simulink model "pixhawkController"  (R2016b)
settings: Solver=FixedStepDiscrete  StartTime=0.0  StopTime=inf  FixedStep=0.01  RelTol=1e-3  EnableMultiTasking=on
undefined symbols (not defined in the file): dt_pixhawk, KiPitchAttitude, KiPitchRate, KiRollAttitude, KiRollRate, KiYawRate, KpPitchAttitude, KpPitchRate, KpRollAttitude, KpRollRate, KpYawRate, PX4_TUNE_ENUM, RGBLED_COLOR_ENUM, RGBLED_MODE_ENUM
libraries: xpcutilitieslib x32, simulink x11, pixhawk_slib_sensors_actuators x8, pixhawk_slib_ADC_serial x2
settings Model: Creator=darenlee  LastModifiedBy=ers
settings DataIOCC: LimitDataPoints=on  SaveFormat=StructureWithTime
settings OptimizationCC: DefaultParameterBehavior=Inlined  LifeSpan=1  MaxStackSize=64
settings DebuggingCC: AllowSymbolicDim=off  SFUnexpectedBacktrackingDiag=warning  SFNoUnconditionalDefaultTransitionDiag=warning  SFExecutionAtInitializationDiag=none
settings HardwareCC: ProdBitPerPointer=32  ProdBitPerSizeT=32  ProdBitPerPtrDiffT=32  ProdLargestAtomicInteger=Long  ProdLargestAtomicFloat=Double  ProdIntDivRoundTo=Undefined  ProdWordSize=32  ProdHWDeviceType=ARM Compatible->ARM Cortex
settings ModelReferenceCC: PropagateSignalLabelsOutOfModel=off
settings RTWCC: SystemTargetFile=ert.tlc  HardwareBoard=Pixhawk PX4  TLCOptions=-aInlineSetEventsForThisBaseRateFcn=TLC_FALSE -aSuppressMultiTaskScheduler=TLC_FALSE -aRateBasedStepFcn=0  TemplateMakefile=ert_default_tmf  Description=Embedded Coder  GenerateReport=on  Toolchain=Pixhawk Toolchain  IncludeHyperlinkInReport=on  LaunchReport=on  GenerateTraceInfo=on  GenerateTraceReport=on  GenerateTraceReportSl=on  GenerateTraceReportSf=on  GenerateTraceReportEml=on
settings CodeAppCC: IgnoreCustomStorageClasses=off
settings ERTTargetCC: ExtModeTransport=1  ExtModeMexFile=ext_serial_win32_comm  ExtModeMexArgs=1 11 115200 5  ERTCustomFileTemplate=PX4_codertarget_file_process.tlc  ConvertIfToSwitch=off  SuppressUnreachableDefaultCases=off
settings ConfigComp: CovMetricSettings=dw  CovHtmlReporting=on  CovSaveCumulativeToWorkspaceVar=on  CovSaveSingleToWorkspaceVar=on  CovExternalEMLEnable=off

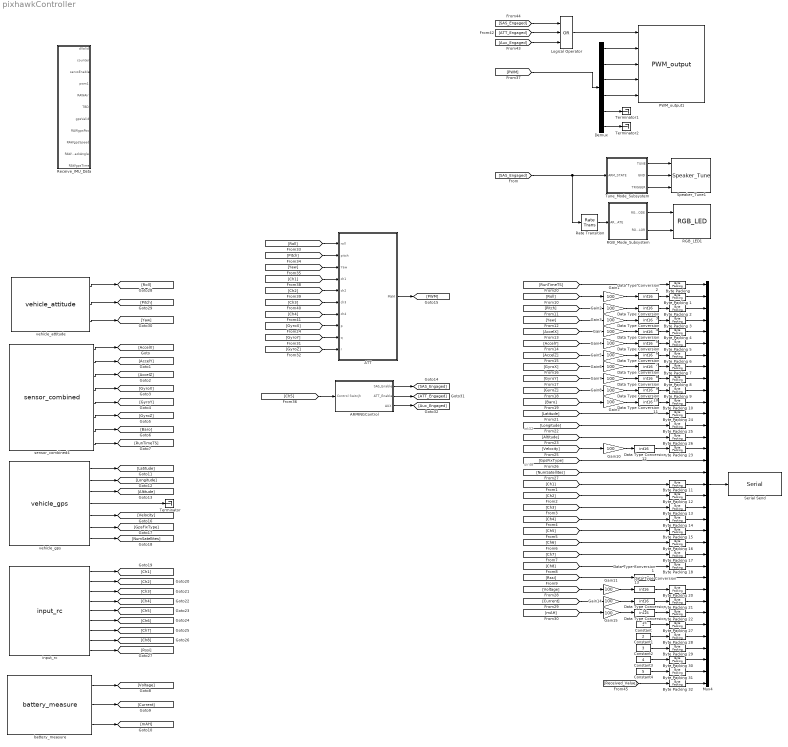
== system pixhawkController ==
  note: uint8
  note: int32
  ARMINGControl : Subsystem
  ATT : Subsystem
  Byte Packing {,1..18,20..32} (32 alike) : xpcutilitieslib/Byte Packing 
  Constant : Constant  OutDataTypeStr=int16
  Constant1 : Constant  Value=2  OutDataTypeStr=int16
  Constant2 : Constant  Value=3  OutDataTypeStr=int16
  Constant3 : Constant  Value=4  OutDataTypeStr=int16
  Constant4 : Constant  Value=5  OutDataTypeStr=int16
  Data Type Conversion1 : DataTypeConversion  OutDataTypeStr=uint8
  Data Type Conversion{2..15} (14 alike) : DataTypeConversion  OutDataTypeStr=int16
  Demux : Demux  Outputs=6
  Gain{,1..11,14..15} (14 alike) : Gain  Gain=100
  Logical Operator : Logic  Operator=OR  Inputs=3  AllPortsSameDT=off  OutDataTypeStr=boolean
  Mux4 : Mux  Inputs=35
  PWM_output1 : pixhawk_slib_sensors_actuators/PWM_output  pwm_rate=50Hz  show_pwm1=on  show_pwm2=on  show_pwm3=on  show_pwm4=on  show_pwm5=off  show_pwm6=off  show_pwm7=off  show_pwm8=off
  RGB_LED1 : pixhawk_slib_sensors_actuators/RGB_LED
  RGB_Mode_Subsystem : Subsystem
  Rate Transition : RateTransition  OutPortSampleTime=1/2
  Receive_IMU_Data : Subsystem
  Serial Send : pixhawk_slib_ADC_serial/Serial  DeviceName=/dev/ttyS5  ReadOrWrite=Writing  BaudRateStr=115200  block=off  WriteStatus=on  Terminator=off  Header=on  NumBytesRead=4  TerminatorChar=\n  HeaderData=[ uint8( hex2dec( '41' ) ), uint8( hex2dec( '42' ) ), uint8( hex2dec( '43' ) ), uint8( hex2dec( '41' ) ) ]  SimulateUsing=Code generation
  Speaker_Tune1 : pixhawk_slib_sensors_actuators/Speaker_Tune
  Terminator : Terminator
  Terminator1 : Terminator
  Terminator2 : Terminator
  Tune_Mode_Subsystem : Subsystem
  battery_measure : pixhawk_slib_sensors_actuators/battery_measure  SampleTime=dt_pixhawk  VoltageOut=on  VoltageFilteredOut=off  CurrentOut=on  mAH_Out=on  TimeStamp=off
  input_rc : pixhawk_slib_sensors_actuators/input_rc  sampletime=dt_pixhawk  channel1=on  channel2=on  channel3=on  channel4=on  channel5=on  channel6=on  channel7=on  channel8=on  ch_count=off  rssi=on  rc_failsafe=off  rc_lost=off  rc_inputsource=off
  sensor_combined4 : pixhawk_slib_sensors_actuators/sensor_combined  sampletime=dt_pixhawk  show_mag=off  show_acc=on  show_gyro=on  show_baro=on  show_ts=on
  vehicle_attitude : pixhawk_slib_sensors_actuators/vehicle_attitude  sampletime=dt_pixhawk  show_r=on  show_p=on  show_y=on  show_q=off
  vehicle_gps : pixhawk_slib_sensors_actuators/vehicle_gps  sampletime=1/100  show_ts_pos=off  show_alt=on  show_ts_gps=off  show_vel=on  show_fixtype=on  show_numsat=on
  wires:
  sensor_combined4/8 -> [RunTimeTS]
  battery_measure/1 -> [Voltage]
  battery_measure/3 -> [mAH]
  battery_measure/2 -> [Current]
  vehicle_gps/2 -> [Longitude]
  vehicle_gps/1 -> [Latitude]
  vehicle_gps/3 -> [Altitude]
  input_rc/2 -> [Ch2]
  input_rc/3 -> [Ch3]
  input_rc/6 -> [Ch6]
  input_rc/8 -> [Ch8]
  input_rc/7 -> [Ch7]
  input_rc/5 -> [Ch5]
  input_rc/4 -> [Ch4]
  input_rc/1 -> [Ch1]
  input_rc/9 -> [Rssi]
  vehicle_attitude/1 -> [Roll]
  vehicle_attitude/2 -> [Pitch]
  vehicle_attitude/3 -> [Yaw]
  vehicle_gps/6 -> [GpsFixType]
  vehicle_gps/5 -> [Velocity]
  vehicle_gps/7 -> [NumSatellites]
  vehicle_gps/4 -> Terminator/1
  "Byte Packing "/1 -> Mux4/1
  [Pitch] -> Gain2/1
  Mux4/1 -> Serial Send/1
  Byte Packing 1/1 -> Mux4/2
  Byte Packing 2/1 -> Mux4/3
  Byte Packing 3/1 -> Mux4/4
  sensor_combined4/4 -> [GyroX]
  sensor_combined4/3 -> [AccelZ]
  sensor_combined4/5 -> [GyroY]
  sensor_combined4/2 -> [AccelY]
  sensor_combined4/6 -> [GyroZ]
  sensor_combined4/7 -> [Baro]
  sensor_combined4/1 -> [AccelX]
  [AccelX] -> Gain/1
  [AccelY] -> Gain4/1
  [AccelZ] -> Gain5/1
  [GyroX] -> Gain6/1
  [GyroY] -> Gain7/1
  [GyroZ] -> Gain8/1
  [Baro] -> Gain9/1
  [Ch1] -> Byte Packing 11/1
  [Ch2] -> Byte Packing 12/1
  [Ch3] -> Byte Packing 13/1
  [Ch4] -> Byte Packing 14/1
  [Ch5] -> Byte Packing 15/1
  [Ch6] -> Byte Packing 16/1
  [Ch7] -> Byte Packing 17/1
  [Ch8] -> Byte Packing 18/1
  [Rssi] -> Data Type Conversion1/1
  [mAH] -> Gain15/1
  [Current] -> Gain14/1
  [Voltage] -> Gain11/1
  [RunTimeTS] -> "Byte Packing "/1
  [Roll] -> Gain1/1
  Data Type Conversion3/1 -> Byte Packing 2/1
  [Yaw] -> Gain3/1
  Data Type Conversion4/1 -> Byte Packing 3/1
  Data Type Conversion2/1 -> Byte Packing 1/1
  Gain1/1 -> Data Type Conversion2/1
  Gain2/1 -> Data Type Conversion3/1
  Gain3/1 -> Data Type Conversion4/1
  Gain/1 -> Data Type Conversion5/1
  Gain4/1 -> Data Type Conversion6/1
  Gain5/1 -> Data Type Conversion7/1
  Gain6/1 -> Data Type Conversion8/1
  Gain7/1 -> Data Type Conversion9/1
  Gain8/1 -> Data Type Conversion10/1
  Gain9/1 -> Data Type Conversion11/1
  Data Type Conversion5/1 -> Byte Packing 4/1
  Data Type Conversion6/1 -> Byte Packing 5/1
  Data Type Conversion7/1 -> Byte Packing 6/1
  Data Type Conversion8/1 -> Byte Packing 7/1
  Data Type Conversion9/1 -> Byte Packing 8/1
  Data Type Conversion10/1 -> Byte Packing 9/1
  Data Type Conversion11/1 -> Byte Packing 10/1
  [Velocity] -> Gain10/1
  Gain10/1 -> Data Type Conversion12/1
  Data Type Conversion12/1 -> Byte Packing 23/1
  [Latitude] -> Byte Packing 24/1
  [Longitude] -> Byte Packing 25/1
  [Altitude] -> Byte Packing 26/1
  [GpsFixType] -> Mux4/16
  [NumSatellites] -> Mux4/17
  Gain11/1 -> Data Type Conversion13/1
  Gain14/1 -> Data Type Conversion14/1
  Gain15/1 -> Data Type Conversion15/1
  Data Type Conversion13/1 -> Byte Packing 20/1
  Data Type Conversion14/1 -> Byte Packing 21/1
  Data Type Conversion15/1 -> Byte Packing 22/1
  Byte Packing 4/1 -> Mux4/5
  Byte Packing 5/1 -> Mux4/6
  Byte Packing 6/1 -> Mux4/7
  Byte Packing 7/1 -> Mux4/8
  Byte Packing 8/1 -> Mux4/9
  Byte Packing 9/1 -> Mux4/10
  Byte Packing 10/1 -> Mux4/11
  Byte Packing 25/1 -> Mux4/13
  Byte Packing 26/1 -> Mux4/14
  Byte Packing 24/1 -> Mux4/12
  Byte Packing 23/1 -> Mux4/15
  Byte Packing 11/1 -> Mux4/18
  Byte Packing 12/1 -> Mux4/19
  Byte Packing 13/1 -> Mux4/20
  Byte Packing 14/1 -> Mux4/21
  Byte Packing 15/1 -> Mux4/22
  Byte Packing 16/1 -> Mux4/23
  Byte Packing 17/1 -> Mux4/24
  Byte Packing 18/1 -> Mux4/25
  Data Type Conversion1/1 -> Mux4/26
  Byte Packing 20/1 -> Mux4/27
  Byte Packing 21/1 -> Mux4/28
  Byte Packing 22/1 -> Mux4/29
  Constant/1 -> Byte Packing 27/1
  Byte Packing 32/1 -> Mux4/35
  Byte Packing 27/1 -> Mux4/30
  Byte Packing 30/1 -> Mux4/33
  Byte Packing 28/1 -> Mux4/31
  Byte Packing 31/1 -> Mux4/34
  Byte Packing 29/1 -> Mux4/32
  Constant1/1 -> Byte Packing 28/1
  Constant2/1 -> Byte Packing 29/1
  Constant3/1 -> Byte Packing 30/1
  Constant4/1 -> Byte Packing 31/1
  RGB_Mode_Subsystem/1(RGB_MODE) -> RGB_LED1/1
  RGB_Mode_Subsystem/2(RGB_COLOR) -> RGB_LED1/2
  Tune_Mode_Subsystem/1(TUNE) -> Speaker_Tune1/1
  Tune_Mode_Subsystem/2(GND) -> Speaker_Tune1/2
  Tune_Mode_Subsystem/3(TRIGGER) -> Speaker_Tune1/3
  [SAS_Engaged] -> Tune_Mode_Subsystem/1(ARM_STATE), Rate Transition/1
  ATT/1(PWM) -> [PWM]
  [Roll] -> ATT/1(roll)
  [Pitch] -> ATT/2(pitch)
  [Yaw] -> ATT/3(Yaw)
  [Ch4] -> ATT/7(ch4)
  [Ch3] -> ATT/6(ch3)
  [Ch2] -> ATT/5(ch2)
  [Ch1] -> ATT/4(ch1)
  [GyroX] -> ATT/8(p)
  [GyroY] -> ATT/9(q)
  [GyroZ] -> ATT/10(r)
  Demux/3 -> PWM_output1/4
  Demux/4 -> PWM_output1/5
  Demux/2 -> PWM_output1/3
  Demux/1 -> PWM_output1/2
  [Ch5] -> ARMINGControl/1(Control Switcjh)
  ARMINGControl/1(SAS_Enable) -> [SAS_Engaged]
  ARMINGControl/2(ATT_Enable) -> [ATT_Engaged]
  ARMINGControl/3(AUX) -> [Aux_Engaged]
  [SAS_Engaged] -> Logical Operator/1
  [ATT_Engaged] -> Logical Operator/2
  [Aux_Engaged] -> Logical Operator/3
  Logical Operator/1 -> PWM_output1/1
  [Received_Value] -> Byte Packing 32/1
  [PWM] -> Demux/1
  Demux/5 -> Terminator1/1
  Demux/6 -> Terminator2/1
  Rate Transition/1 -> RGB_Mode_Subsystem/1(ARM_STATE)

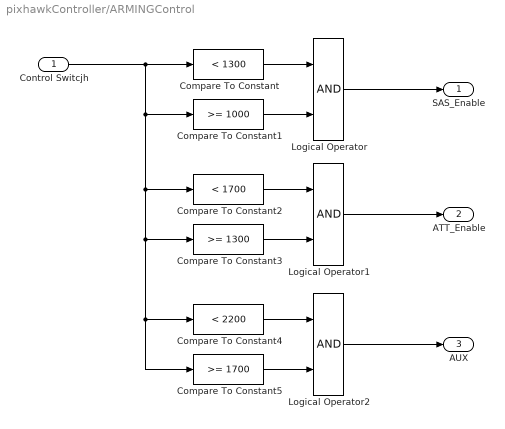
== system pixhawkController/ARMINGControl ==
  Control Switcjh : Inport
  Compare To Constant : simulink/Logic and Bit Operations/Compare To Constant  relop=<  const=1300  OutDataTypeStr=boolean
  Compare To Constant1 : simulink/Logic and Bit Operations/Compare To Constant  relop=>=  const=1000  OutDataTypeStr=boolean
  Compare To Constant2 : simulink/Logic and Bit Operations/Compare To Constant  relop=<  const=1700  OutDataTypeStr=boolean
  Compare To Constant3 : simulink/Logic and Bit Operations/Compare To Constant  relop=>=  const=1300  OutDataTypeStr=boolean
  Compare To Constant4 : simulink/Logic and Bit Operations/Compare To Constant  relop=<  const=2200  OutDataTypeStr=boolean
  Compare To Constant5 : simulink/Logic and Bit Operations/Compare To Constant  relop=>=  const=1700  OutDataTypeStr=boolean
  Logical Operator : Logic  AllPortsSameDT=off  OutDataTypeStr=boolean
  Logical Operator1 : Logic  AllPortsSameDT=off  OutDataTypeStr=boolean
  Logical Operator2 : Logic  AllPortsSameDT=off  OutDataTypeStr=boolean
  SAS_Enable : Outport
  ATT_Enable : Outport  Port=2
  AUX : Outport  Port=3
  wires:
  Control Switcjh/1 -> Compare To Constant5/1, Compare To Constant4/1, Compare To Constant3/1, Compare To Constant2/1, Compare To Constant1/1, Compare To Constant/1
  Compare To Constant/1 -> Logical Operator/1
  Compare To Constant1/1 -> Logical Operator/2
  Logical Operator/1 -> SAS_Enable/1
  Compare To Constant2/1 -> Logical Operator1/1
  Compare To Constant3/1 -> Logical Operator1/2
  Logical Operator1/1 -> ATT_Enable/1
  Compare To Constant4/1 -> Logical Operator2/1
  Compare To Constant5/1 -> Logical Operator2/2
  Logical Operator2/1 -> AUX/1

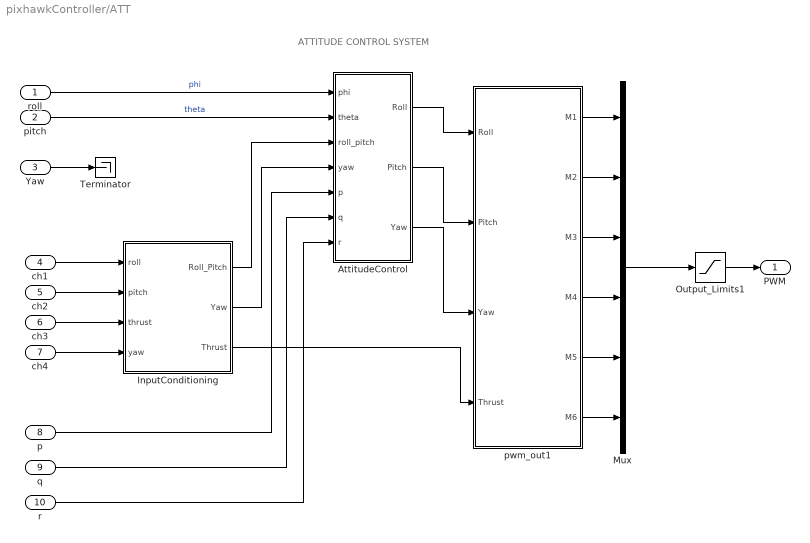
== system pixhawkController/ATT ==
  note: ATTITUDE CONTROL SYSTEM
  roll : Inport  OutDataTypeStr=single  PortDimensions=1
  pitch : Inport  Port=2  PortDimensions=1
  Yaw : Inport  Port=3  PortDimensions=1
  ch1 : Inport  Port=4  OutDataTypeStr=uint16  PortDimensions=1
  ch2 : Inport  Port=5  OutDataTypeStr=uint16  PortDimensions=1
  ch3 : Inport  Port=6  OutDataTypeStr=uint16  PortDimensions=1
  ch4 : Inport  Port=7  OutDataTypeStr=uint16  PortDimensions=1
  p : Inport  Port=8  PortDimensions=1
  q : Inport  Port=9  PortDimensions=1
  r : Inport  Port=10  PortDimensions=1
  AttitudeControl : Subsystem
  InputConditioning : Subsystem
  Mux : Mux  Inputs=6
  Output_Limits1 : Saturate  UpperLimit=2000  LowerLimit=1000
  Terminator : Terminator
  pwm_out1 : MATLAB Function  TreatAsAtomicUnit=on  SystemSampleTime=dt_pixhawk
  PWM : Outport  PortDimensions=6
  wires:
  Mux/1 -> Output_Limits1/1
  Output_Limits1/1 -> PWM/1
  InputConditioning/3(Thrust) -> pwm_out1/4(Thrust)
  roll/1 -> AttitudeControl/1(phi)  "phi"
  pitch/1 -> AttitudeControl/2(theta)  "theta"
  InputConditioning/1(Roll_Pitch) -> AttitudeControl/3(roll_pitch)
  InputConditioning/2(Yaw) -> AttitudeControl/4(yaw)
  p/1 -> AttitudeControl/5(p)
  q/1 -> AttitudeControl/6(q)
  r/1 -> AttitudeControl/7(r)
  AttitudeControl/1(Roll) -> pwm_out1/1(Roll)
  AttitudeControl/2(Pitch) -> pwm_out1/2(Pitch)
  AttitudeControl/3(Yaw) -> pwm_out1/3(Yaw)
  ch1/1 -> InputConditioning/1(roll)
  ch2/1 -> InputConditioning/2(pitch)
  ch4/1 -> InputConditioning/4(yaw)
  ch3/1 -> InputConditioning/3(thrust)
  Yaw/1 -> Terminator/1
  pwm_out1/4(M4) -> Mux/4
  pwm_out1/3(M3) -> Mux/3
  pwm_out1/2(M2) -> Mux/2
  pwm_out1/1(M1) -> Mux/1
  pwm_out1/5(M5) -> Mux/5
  pwm_out1/6(M6) -> Mux/6

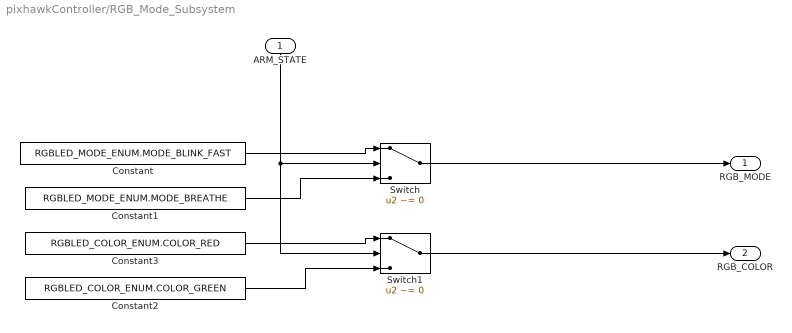
== system pixhawkController/RGB_Mode_Subsystem ==
  ARM_STATE : Inport
  Constant : Constant  Value=RGBLED_MODE_ENUM.MODE_BLINK_FAST  OutDataTypeStr=Enum: RGBLED_MODE_ENUM
  Constant1 : Constant  Value=RGBLED_MODE_ENUM.MODE_BREATHE  OutDataTypeStr=Enum: RGBLED_MODE_ENUM
  Constant2 : Constant  Value=RGBLED_COLOR_ENUM.COLOR_GREEN  OutDataTypeStr=Enum: RGBLED_COLOR_ENUM
  Constant3 : Constant  Value=RGBLED_COLOR_ENUM.COLOR_RED  OutDataTypeStr=Enum: RGBLED_COLOR_ENUM
  Switch : Switch  Criteria=u2 ~= 0  Threshold=1500  SampleTime=1/2
  Switch1 : Switch  Criteria=u2 ~= 0  Threshold=1500  SampleTime=1/2
  RGB_MODE : Outport
  RGB_COLOR : Outport  Port=2
  wires:
  ARM_STATE/1 -> Switch1/2, Switch/2
  Constant/1 -> Switch/1
  Constant1/1 -> Switch/3
  Switch/1 -> RGB_MODE/1
  Constant3/1 -> Switch1/1
  Constant2/1 -> Switch1/3
  Switch1/1 -> RGB_COLOR/1

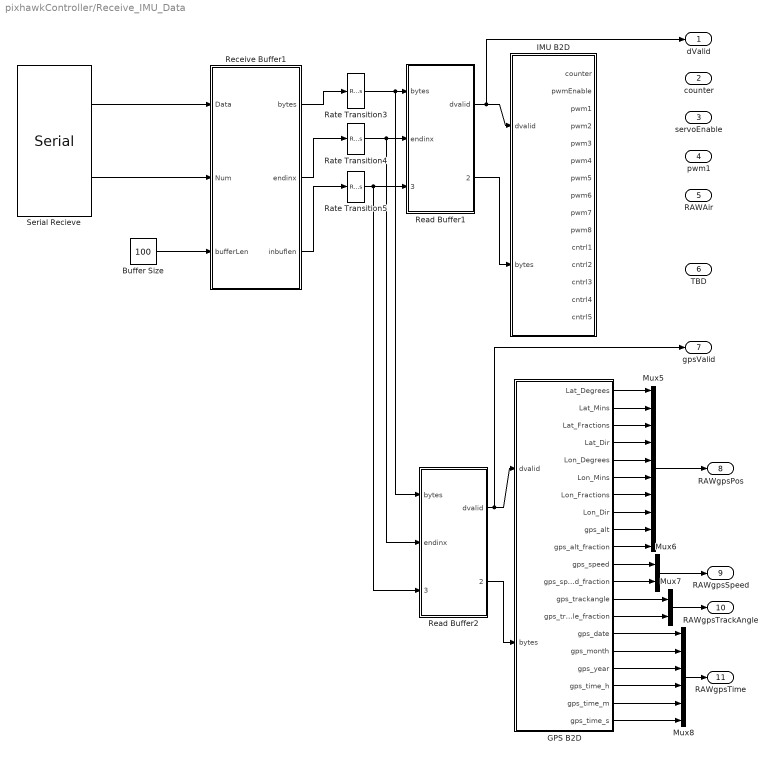
== system pixhawkController/Receive_IMU_Data ==
  Buffer Size : Constant  Value=100
  GPS B2D : MATLAB Function  TreatAsAtomicUnit=on
  IMU B2D : MATLAB Function  TreatAsAtomicUnit=on
  Mux5 : Mux  Inputs=10
  Mux6 : Mux  Inputs=2
  Mux7 : Mux  Inputs=2
  Mux8 : Mux  Inputs=6
  Rate Transition3 : RateTransition  OutPortSampleTime=dt
  Rate Transition4 : RateTransition  OutPortSampleTime=dt
  Rate Transition5 : RateTransition  OutPortSampleTime=dt
  Read Buffer1 : MATLAB Function  TreatAsAtomicUnit=on
  Read Buffer2 : MATLAB Function  TreatAsAtomicUnit=on
  Receive Buffer1 : MATLAB Function  TreatAsAtomicUnit=on
  Serial Recieve : pixhawk_slib_ADC_serial/Serial  DeviceName=/dev/ttyS5  ReadOrWrite=Reading  BaudRateStr=115200  block=off  WriteStatus=on  Terminator=off  Header=off  NumBytesRead=4  TerminatorChar=\n  HeaderData=[ uint8( hex2dec( 'DE' ) ), uint8( hex2dec( 'AD' ) ), uint8( hex2dec( 'C0' ) ), uint8( hex2dec( 'DE' ) ) ]  SimulateUsing=Code generation
  dValid : Outport
  counter : Outport  Port=2
  servoEnable : Outport  Port=3
  pwm1 : Outport  Port=4
  RAWAir : Outport  Port=5
  TBD : Outport  Port=6
  gpsValid : Outport  Port=7
  RAWgpsPos : Outport  Port=8
  RAWgpsSpeed : Outport  Port=9
  RAWgpsTrackAngle : Outport  Port=10
  RAWgpsTime : Outport  Port=11
  wires:
  Rate Transition3/1 -> Read Buffer1/1(bytes), Read Buffer2/1(bytes)
  Receive Buffer1/1(bytes) -> Rate Transition3/1
  Receive Buffer1/2(endinx) -> Rate Transition4/1
  Receive Buffer1/3(inbuflen) -> Rate Transition5/1
  Rate Transition4/1 -> Read Buffer1/2(endinx), Read Buffer2/2(endinx)
  Rate Transition5/1 -> Read Buffer1/3(inbuflenSC2), Read Buffer2/3(inbuflenSC2)
  Serial Recieve/1 -> Receive Buffer1/1(Data)
  Serial Recieve/2 -> Receive Buffer1/2(Num)
  Read Buffer1/1(dvalid) -> IMU B2D/1(dvalid), dValid/1
  Read Buffer1/2(imu_data) -> IMU B2D/2(bytes)
  Read Buffer2/1(dvalid) -> gpsValid/1, GPS B2D/1(dvalid)
  Read Buffer2/2(imu_data) -> GPS B2D/2(bytes)
  GPS B2D/1(Lat_Degrees) -> Mux5/1
  GPS B2D/2(Lat_Mins) -> Mux5/2
  GPS B2D/3(Lat_Fractions) -> Mux5/3
  GPS B2D/4(Lat_Dir) -> Mux5/4
  GPS B2D/5(Lon_Degrees) -> Mux5/5
  GPS B2D/6(Lon_Mins) -> Mux5/6
  GPS B2D/7(Lon_Fractions) -> Mux5/7
  GPS B2D/8(Lon_Dir) -> Mux5/8
  GPS B2D/9(gps_alt) -> Mux5/9
  GPS B2D/10(gps_alt_fraction) -> Mux5/10
  Mux5/1 -> RAWgpsPos/1
  GPS B2D/11(gps_speed) -> Mux6/1
  GPS B2D/12(gps_speed_fraction) -> Mux6/2
  Mux6/1 -> RAWgpsSpeed/1
  GPS B2D/13(gps_trackangle) -> Mux7/1
  GPS B2D/14(gps_trackangle_fraction) -> Mux7/2
  Mux7/1 -> RAWgpsTrackAngle/1
  GPS B2D/15(gps_date) -> Mux8/1
  GPS B2D/16(gps_month) -> Mux8/2
  GPS B2D/17(gps_year) -> Mux8/3
  GPS B2D/18(gps_time_h) -> Mux8/4
  GPS B2D/19(gps_time_m) -> Mux8/5
  GPS B2D/20(gps_time_s) -> Mux8/6
  Mux8/1 -> RAWgpsTime/1
  Buffer Size/1 -> Receive Buffer1/3(bufferLen)

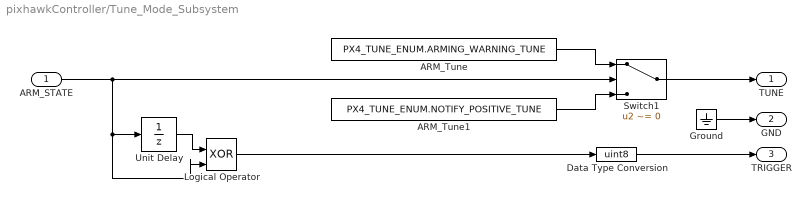
== system pixhawkController/Tune_Mode_Subsystem ==
  ARM_STATE : Inport
  ARM_Tune : Constant  Value=PX4_TUNE_ENUM.ARMING_WARNING_TUNE  OutDataTypeStr=Enum: PX4_TUNE_ENUM
  ARM_Tune1 : Constant  Value=PX4_TUNE_ENUM.NOTIFY_POSITIVE_TUNE  OutDataTypeStr=Enum: PX4_TUNE_ENUM
  Data Type Conversion : DataTypeConversion  OutDataTypeStr=uint8
  Ground : Ground
  Logical Operator : Logic  Operator=XOR  IconShape=distinctive  AllPortsSameDT=off  OutDataTypeStr=boolean
  Switch1 : Switch  Criteria=u2 ~= 0  Threshold=1500
  Unit Delay : UnitDelay  SampleTime=-1
  TUNE : Outport
  GND : Outport  Port=2
  TRIGGER : Outport  Port=3
  wires:
  Ground/1 -> GND/1
  Data Type Conversion/1 -> TRIGGER/1
  Switch1/1 -> TUNE/1
  ARM_Tune/1 -> Switch1/1
  ARM_Tune1/1 -> Switch1/3
  ARM_STATE/1 -> Logical Operator/2, Unit Delay/1, Switch1/2
  Unit Delay/1 -> Logical Operator/1
  Logical Operator/1 -> Data Type Conversion/1

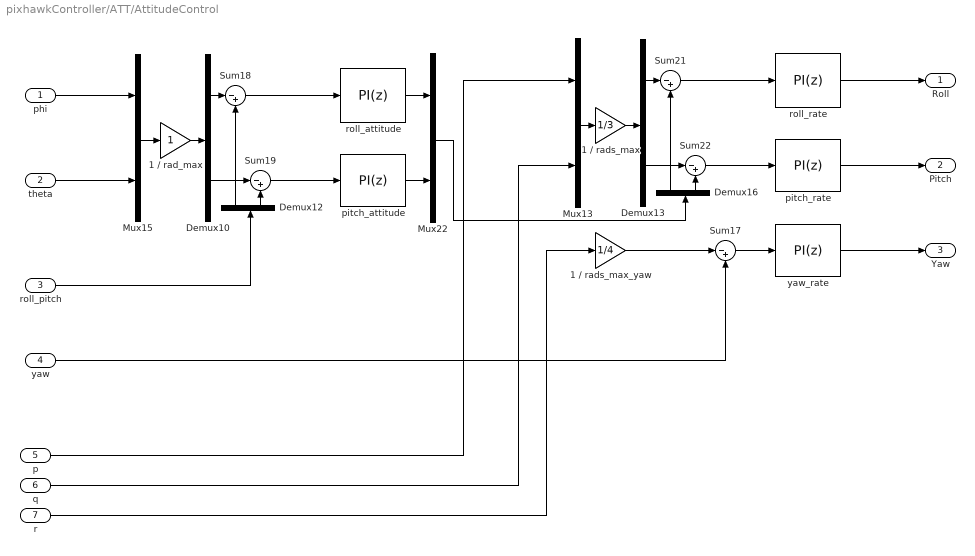
== system pixhawkController/ATT/AttitudeControl ==
  phi : Inport
  theta : Inport  Port=2
  roll_pitch : Inport  Port=3
  yaw : Inport  Port=4
  p : Inport  Port=5
  q : Inport  Port=6
  r : Inport  Port=7
  1 / rad_max : Gain
  1 / rads_max : Gain  Gain=1/3
  1 / rads_max_yaw : Gain  Gain=1/4
  Demux{10,12..13,16} (4 alike) : Demux  Outputs=2
  Mux13 : Mux  Inputs=2
  Mux15 : Mux  Inputs=2
  Mux22 : Mux  Inputs=2
  Sum{17..19,21..22} (5 alike) : Sum  Inputs=|-+
  pitch_attitude : simulink/Continuous/PID Controller  Controller=PI  TimeDomain=Discrete-time  SampleTime=-1  IntegratorMethod=Forward Euler  FilterMethod=Forward Euler  Form=Parallel  UseFilter=on  ControllerParametersSource=internal  P=KpPitchAttitude  I=KiPitchAttitude  D=0.01  N=100  InitialConditionSource=internal  InitialConditionForIntegrator=0  InitialConditionForFilter=0  ExternalReset=none  LimitOutput=on  UpperSaturationLimit=1  LowerSaturationLimit=-1  LinearizeAsGain=on  AntiWindupMode=back-calculation  Kb=1  TrackingMode=off  Kt=1  PParamMin=[]  PParamMax=[]  IParamMin=[]  IParamMax=[]  DParamMin=[]  DParamMax=[]  NParamMin=[]  NParamMax=[]  KbParamMin=[]  KbParamMax=[]  KtParamMin=[]  KtParamMax=[]  POutMin=[]  POutMax=[]  IOutMin=[]  IOutMax=[]  DOutMin=[]  DOutMax=[]  NOutMin=[]  NOutMax=[]  KbOutMin=[]  KbOutMax=[]  KtOutMin=[]  KtOutMax=[]  IntegratorOutMin=[]  IntegratorOutMax=[]  FilterOutMin=[]  FilterOutMax=[]  SumOutMin=[]  SumOutMax=[]  SumI1OutMin=[]  SumI1OutMax=[]  SumI2OutMin=[]  SumI2OutMax=[]  SumI3OutMin=[]  SumI3OutMax=[]  SumDOutMin=[]  SumDOutMax=[]  SaturationOutMin=[]  SaturationOutMax=[]  IntegratorContinuousStateAttributes=''  IntegratorStateMustResolveToSignalObject=off  IntegratorRTWStateStorageClass=Auto  FilterContinuousStateAttributes=''  FilterStateMustResolveToSignalObject=off  FilterRTWStateStorageClass=Auto  DifferentiatorICPrevScaledInput=0  DifferentiatorOutMin=[]  DifferentiatorOutMax=[]
  pitch_rate : simulink/Continuous/PID Controller  Controller=PI  TimeDomain=Discrete-time  SampleTime=-1  IntegratorMethod=Forward Euler  FilterMethod=Forward Euler  Form=Parallel  UseFilter=on  ControllerParametersSource=internal  P=KpPitchRate  I=KiPitchRate  D=0.0024  N=100  InitialConditionSource=internal  InitialConditionForIntegrator=0  InitialConditionForFilter=0  ExternalReset=none  LimitOutput=on  UpperSaturationLimit=1  LowerSaturationLimit=-1  LinearizeAsGain=on  AntiWindupMode=back-calculation  Kb=1  TrackingMode=off  Kt=1  PParamMin=[]  PParamMax=[]  IParamMin=[]  IParamMax=[]  DParamMin=[]  DParamMax=[]  NParamMin=[]  NParamMax=[]  KbParamMin=[]  KbParamMax=[]  KtParamMin=[]  KtParamMax=[]  POutMin=[]  POutMax=[]  IOutMin=[]  IOutMax=[]  DOutMin=[]  DOutMax=[]  NOutMin=[]  NOutMax=[]  KbOutMin=[]  KbOutMax=[]  KtOutMin=[]  KtOutMax=[]  IntegratorOutMin=[]  IntegratorOutMax=[]  FilterOutMin=[]  FilterOutMax=[]  SumOutMin=[]  SumOutMax=[]  SumI1OutMin=[]  SumI1OutMax=[]  SumI2OutMin=[]  SumI2OutMax=[]  SumI3OutMin=[]  SumI3OutMax=[]  SumDOutMin=[]  SumDOutMax=[]  SaturationOutMin=[]  SaturationOutMax=[]  IntegratorContinuousStateAttributes=''  IntegratorStateMustResolveToSignalObject=off  IntegratorRTWStateStorageClass=Auto  FilterContinuousStateAttributes=''  FilterStateMustResolveToSignalObject=off  FilterRTWStateStorageClass=Auto  DifferentiatorICPrevScaledInput=0  DifferentiatorOutMin=[]  DifferentiatorOutMax=[]
  roll_attitude : simulink/Continuous/PID Controller  Controller=PI  TimeDomain=Discrete-time  SampleTime=-1  IntegratorMethod=Forward Euler  FilterMethod=Forward Euler  Form=Parallel  UseFilter=on  ControllerParametersSource=internal  P=KpRollAttitude  I=KiRollAttitude  D=0.01  N=100  InitialConditionSource=internal  InitialConditionForIntegrator=0  InitialConditionForFilter=0  ExternalReset=none  LimitOutput=on  UpperSaturationLimit=1  LowerSaturationLimit=-1  LinearizeAsGain=on  AntiWindupMode=back-calculation  Kb=1  TrackingMode=off  Kt=1  PParamMin=[]  PParamMax=[]  IParamMin=[]  IParamMax=[]  DParamMin=[]  DParamMax=[]  NParamMin=[]  NParamMax=[]  KbParamMin=[]  KbParamMax=[]  KtParamMin=[]  KtParamMax=[]  POutMin=[]  POutMax=[]  IOutMin=[]  IOutMax=[]  DOutMin=[]  DOutMax=[]  NOutMin=[]  NOutMax=[]  KbOutMin=[]  KbOutMax=[]  KtOutMin=[]  KtOutMax=[]  IntegratorOutMin=[]  IntegratorOutMax=[]  FilterOutMin=[]  FilterOutMax=[]  SumOutMin=[]  SumOutMax=[]  SumI1OutMin=[]  SumI1OutMax=[]  SumI2OutMin=[]  SumI2OutMax=[]  SumI3OutMin=[]  SumI3OutMax=[]  SumDOutMin=[]  SumDOutMax=[]  SaturationOutMin=[]  SaturationOutMax=[]  IntegratorContinuousStateAttributes=''  IntegratorStateMustResolveToSignalObject=off  IntegratorRTWStateStorageClass=Auto  FilterContinuousStateAttributes=''  FilterStateMustResolveToSignalObject=off  FilterRTWStateStorageClass=Auto  DifferentiatorICPrevScaledInput=0  DifferentiatorOutMin=[]  DifferentiatorOutMax=[]
  roll_rate : simulink/Continuous/PID Controller  Controller=PI  TimeDomain=Discrete-time  SampleTime=-1  IntegratorMethod=Forward Euler  FilterMethod=Forward Euler  Form=Parallel  UseFilter=on  ControllerParametersSource=internal  P=KpRollRate  I=KiRollRate  D=0.0024  N=100  InitialConditionSource=internal  InitialConditionForIntegrator=0  InitialConditionForFilter=0  ExternalReset=none  LimitOutput=on  UpperSaturationLimit=1  LowerSaturationLimit=-1  LinearizeAsGain=on  AntiWindupMode=back-calculation  Kb=1  TrackingMode=off  Kt=1  PParamMin=[]  PParamMax=[]  IParamMin=[]  IParamMax=[]  DParamMin=[]  DParamMax=[]  NParamMin=[]  NParamMax=[]  KbParamMin=[]  KbParamMax=[]  KtParamMin=[]  KtParamMax=[]  POutMin=[]  POutMax=[]  IOutMin=[]  IOutMax=[]  DOutMin=[]  DOutMax=[]  NOutMin=[]  NOutMax=[]  KbOutMin=[]  KbOutMax=[]  KtOutMin=[]  KtOutMax=[]  IntegratorOutMin=[]  IntegratorOutMax=[]  FilterOutMin=[]  FilterOutMax=[]  SumOutMin=[]  SumOutMax=[]  SumI1OutMin=[]  SumI1OutMax=[]  SumI2OutMin=[]  SumI2OutMax=[]  SumI3OutMin=[]  SumI3OutMax=[]  SumDOutMin=[]  SumDOutMax=[]  SaturationOutMin=[]  SaturationOutMax=[]  IntegratorContinuousStateAttributes=''  IntegratorStateMustResolveToSignalObject=off  IntegratorRTWStateStorageClass=Auto  FilterContinuousStateAttributes=''  FilterStateMustResolveToSignalObject=off  FilterRTWStateStorageClass=Auto  DifferentiatorICPrevScaledInput=0  DifferentiatorOutMin=[]  DifferentiatorOutMax=[]
  yaw_rate : simulink/Continuous/PID Controller  Controller=PI  TimeDomain=Discrete-time  SampleTime=-1  IntegratorMethod=Forward Euler  FilterMethod=Forward Euler  Form=Parallel  UseFilter=on  ControllerParametersSource=internal  P=KpYawRate  I=KiYawRate  D=0  N=100  InitialConditionSource=internal  InitialConditionForIntegrator=0  InitialConditionForFilter=0  ExternalReset=none  LimitOutput=on  UpperSaturationLimit=1  LowerSaturationLimit=-1  LinearizeAsGain=on  AntiWindupMode=back-calculation  Kb=1  TrackingMode=off  Kt=1  PParamMin=[]  PParamMax=[]  IParamMin=[]  IParamMax=[]  DParamMin=[]  DParamMax=[]  NParamMin=[]  NParamMax=[]  KbParamMin=[]  KbParamMax=[]  KtParamMin=[]  KtParamMax=[]  POutMin=[]  POutMax=[]  IOutMin=[]  IOutMax=[]  DOutMin=[]  DOutMax=[]  NOutMin=[]  NOutMax=[]  KbOutMin=[]  KbOutMax=[]  KtOutMin=[]  KtOutMax=[]  IntegratorOutMin=[]  IntegratorOutMax=[]  FilterOutMin=[]  FilterOutMax=[]  SumOutMin=[]  SumOutMax=[]  SumI1OutMin=[]  SumI1OutMax=[]  SumI2OutMin=[]  SumI2OutMax=[]  SumI3OutMin=[]  SumI3OutMax=[]  SumDOutMin=[]  SumDOutMax=[]  SaturationOutMin=[]  SaturationOutMax=[]  IntegratorContinuousStateAttributes=''  IntegratorStateMustResolveToSignalObject=off  IntegratorRTWStateStorageClass=Auto  FilterContinuousStateAttributes=''  FilterStateMustResolveToSignalObject=off  FilterRTWStateStorageClass=Auto  DifferentiatorICPrevScaledInput=0  DifferentiatorOutMin=[]  DifferentiatorOutMax=[]
  Roll : Outport
  Pitch : Outport  Port=2
  Yaw : Outport  Port=3
  wires:
  r/1 -> 1 / rads_max_yaw/1
  q/1 -> Mux13/2
  Mux22/1 -> Demux16/1
  yaw_rate/1 -> Yaw/1
  phi/1 -> Mux15/1
  Mux15/1 -> 1 / rad_max/1
  theta/1 -> Mux15/2
  1 / rads_max_yaw/1 -> Sum17/1
  roll_rate/1 -> Roll/1
  Sum19/1 -> pitch_attitude/1
  pitch_attitude/1 -> Mux22/2
  roll_attitude/1 -> Mux22/1
  Demux16/1 -> Sum21/2
  yaw/1 -> Sum17/2
  roll_pitch/1 -> Demux12/1
  Demux16/2 -> Sum22/2
  Demux12/1 -> Sum18/2
  Demux12/2 -> Sum19/2
  p/1 -> Mux13/1
  Demux10/1 -> Sum18/1
  Demux10/2 -> Sum19/1
  1 / rad_max/1 -> Demux10/1
  Sum18/1 -> roll_attitude/1
  pitch_rate/1 -> Pitch/1
  Mux13/1 -> 1 / rads_max/1
  Sum22/1 -> pitch_rate/1
  Sum17/1 -> yaw_rate/1
  Demux13/1 -> Sum21/1
  Demux13/2 -> Sum22/1
  1 / rads_max/1 -> Demux13/1
  Sum21/1 -> roll_rate/1

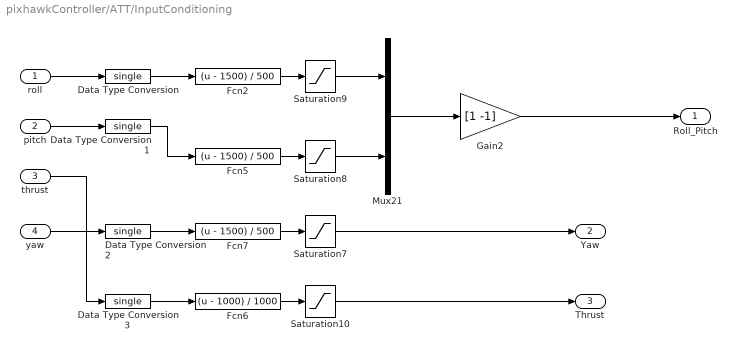
== system pixhawkController/ATT/InputConditioning ==
  roll : Inport
  pitch : Inport  Port=2
  thrust : Inport  Port=3
  yaw : Inport  Port=4
  Data Type Conversion{,1..3} (4 alike) : DataTypeConversion  OutDataTypeStr=single
  Fcn2 : Fcn  Expr=(u - 1500) / 500
  Fcn5 : Fcn  Expr=(u - 1500) / 500
  Fcn6 : Fcn  Expr=(u - 1000) / 1000
  Fcn7 : Fcn  Expr=(u - 1500) / 500
  Gain2 : Gain  Gain=[1 -1]  OutDataTypeStr=Inherit: Inherit via back propagation
  Mux21 : Mux  Inputs=2
  Saturation10 : Saturate  UpperLimit=1  LowerLimit=0
  Saturation7 : Saturate  UpperLimit=1  LowerLimit=-1
  Saturation8 : Saturate  UpperLimit=1  LowerLimit=-1
  Saturation9 : Saturate  UpperLimit=1  LowerLimit=-1
  Roll_Pitch : Outport
  Yaw : Outport  Port=2
  Thrust : Outport  Port=3
  wires:
  Saturation10/1 -> Thrust/1
  Saturation7/1 -> Yaw/1
  Gain2/1 -> Roll_Pitch/1
  Mux21/1 -> Gain2/1
  Saturation8/1 -> Mux21/2
  Fcn6/1 -> Saturation10/1
  thrust/1 -> Data Type Conversion3/1
  Fcn2/1 -> Saturation9/1
  Fcn5/1 -> Saturation8/1
  Saturation9/1 -> Mux21/1
  Fcn7/1 -> Saturation7/1
  yaw/1 -> Data Type Conversion2/1
  pitch/1 -> Data Type Conversion1/1
  roll/1 -> Data Type Conversion/1
  Data Type Conversion/1 -> Fcn2/1
  Data Type Conversion1/1 -> Fcn5/1
  Data Type Conversion2/1 -> Fcn7/1
  Data Type Conversion3/1 -> Fcn6/1

== matlab function pixhawkController/Receive_IMU_Data/IMU B2D ==
  data: dvalid input; counter output uint16; pwmEnable output uint16; pwm1 output uint16; pwm2 output uint16; pwm3 output uint16; pwm4 output uint16; pwm5 output uint16; pwm6 output uint16; pwm7 output uint16; pwm8 output uint16; cntrl1 output uint16; cntrl2 output uint16; bytes input uint8; cntrl3 output; cntrl4 output; cntrl5 output
function [counter, pwmEnable, pwm1, pwm2, pwm3, pwm4, pwm5, pwm6, pwm7, pwm8, cntrl1,cntrl2, cntrl3, cntrl4, cntrl5] = B2D(dvalid,bytes)

persistent counterTemp, pwmEnableTemp, pwm1Temp, pwm2Temp, pwm3Temp, pwm4Temp, pwm5Temp, pwm6Temp, pwm7Temp, pwm8Temp, cntrl1Temp,cntrl2Temp, cntrl3Temp, cntrl4Temp, cntrl5Temp 
% Initialize persistent data
if isempty(counterTemp)
   counterTemp=uint16(0);
end
if isempty(pwm1Temp)
   pwm1Temp=uint16(0);
end
if isempty(pwm2Temp)
   pwm2Temp=uint16(0);
end
if isempty(pwm3Temp)
   pwm3Temp=uint16(0);
end
if isempty(pwm4Temp)
   pwm4Temp=uint16(0);
end
if isempty(pwm5Temp)
   pwm5Temp=uint16(0);
end
if isempty(pwm6Temp)
   pwm6Temp=uint16(0);
end
if isempty(pwm7Temp)
   pwm7Temp=uint16(0);
end
if isempty(pwm8Temp)
   pwm8Temp=uint16(0);
end
if isempty(cntrl1Temp)
   cntrl1Temp=uint16(0);
end
if isempty(cntrl2Temp)
   cntrl2Temp=uint16(0);
end
if isempty(cntrl3Temp)
   cntrl3Temp=uint16(0);
end
if isempty(cntrl4Temp)
   cntrl4Temp=uint16(0);
end
if isempty(cntrl5Temp)
   cntrl5Temp=uint16(0);
end

if (dvalid == 1)
    YaccX= typecast(bytes(2:-1:1),'uint16');
    YaccY= typecast(bytes(4:-1:3),'uint16');
    YaccZ= typecast(bytes(6:-1:5),'uint16');
    YgyroX= typecast(bytes(8:-1:7),'uint16');
    YgyroY= typecast(bytes(10:-1:9),'uint16');
    YgyroZ= typecast(bytes(12:-1:11),'uint16');
    YmagX= typecast(bytes(14:-1:13),'uint16');
    YmagY= typecast(bytes(16:-1:15),'uint16');
    YmagZ= typecast(bytes(18:-1:17),'uint16');
    Ytemp= typecast(bytes(20:-1:19),'uint16');
    Yalt= typecast(bytes(22:-1:21),'uint16');
    Yairs= typecast(bytes(24:-1:23),'uint16');
    Ytemp1= typecast(bytes(26:-1:25),'uint16');
    Ytemp2= typecast(bytes(28:-1:27),'uint16');
    Ytemp3= typecast(bytes(30:-1:29),'uint16');
    Ytemp4= typecast(bytes(32:-1:31),'uint16');
    Ytemp5= typecast(bytes(34:-1:33),'uint16');
    Ytemp6= typecast(bytes(36:-1:35),'uint16');
    Ytemp7= typecast(bytes(38:-1:37),'uint16');
    Ytemp8= typecast(bytes(40:-1:39),'uint16');
    
    XaccX=YaccX(1) ;
    XaccY=YaccY(1) ;
    XaccZ=YaccZ(1) ;
    XgyroX=YgyroX(1);
    XgyroY=YgyroY(1);
    XgyroZ=YgyroZ(1);
    XmagX=YmagX(1);
    XmagY=YmagY(1);
    XmagZ=YmagZ(1); 
    Xtemp=Ytemp(1);
    Xalt=Yalt(1);
    Xairs=Yairs(1);
    Xtemp1=Ytemp1(1);
    Xtemp2=Ytemp2(1);
    Xtemp3=Ytemp3(1);
    Xtemp4=Ytemp4(1);
    Xtemp5=Ytemp5(1);
    Xtemp6=Ytemp6(1);
    Xtemp7=Ytemp7(1);
    Xtemp8=Ytemp8(1);
    
    
end
    
    %ivalue = typecast(bytes(24:-1:23),'uint16');
   accX=XaccX ;
   accY=XaccY ;
   accZ=XaccZ ;
   gyroX=XgyroX;
   gyroY=XgyroY;
   gyroZ=XgyroZ;
   magX=XmagX;
   magY=XmagY;
   magZ=XmagZ; 
   temp=Xtemp;
   alt=Xalt;
   airs=Xairs;
   temp1=Xtemp1;
   temp2=Xtemp2;
   temp3=Xtemp3;
   temp4=Xtemp4;
   temp5=Xtemp5;
   temp6=Xtemp6;
    temp7=Xtemp7;
   temp8=Xtemp8;
   % value = uint8(ivalue(1));
%end

== matlab function pixhawkController/Receive_IMU_Data/Receive Buffer1 ==
  data: Data input uint8; bytes output uint8; endinx output; Num input; inbuflen output; bufferLen input
function [bytes, endinx, inbuflen] = buffer(Data, Num, bufferLen)

persistent rdata inx

% Initialize persistent data
if isempty(rdata)
    rdata = uint8(zeros(bufferLen,1));
end
if isempty(inx)
    inx = 1;
end

% If Data exists
if (Num > 0)
    for inxdata = 1:Num        
        % Grap Data bytes    
        rdata(inx) = Data(inxdata);
        inx = inx + 1;
        if (inx > bufferLen)
            inx = 1;
        end
    end %for
end %if

endinx = inx;
bytes = rdata;
inbuflen = bufferLen;

== matlab function pixhawkController/ATT/pwm_out1 ==
  data: Roll input; M1 output; Pitch input; Yaw input; Thrust input; M2 output; M3 output; M4 output; M5 output; M6 output
function [M1, M2, M3, M4, M5, M6] = motor_mixer(Roll, Pitch, Yaw, Thrust)

%idle_PWM = uint16(1000);

%Quad X
M1 = uint16(0);
M2 = uint16(0);
M3 = uint16(0);
M4 = uint16(0);
M5 = uint16(0);
M6 = uint16(0);
% Quad +
% M1 = ((Pitch - Yaw) * Thrust / 2 + Thrust) * 1000 + idle_PWM;
% M2 = ((-Roll + Yaw) * Thrust / 2 + Thrust) * 1000 + idle_PWM;
% M3 = ((-Pitch - Yaw) * Thrust / 2 + Thrust) * 1000 + idle_PWM;
% M4 = ((Roll + Yaw) * Thrust / 2 + Thrust) * 1000 + idle_PWM;
% M5 = 1000;
% M6 = 1000;
% M7 = 1000;
% M8 = 1000;

% Hex X
% M1 = ((Pitch + Roll / 2 - Yaw) * Thrust / 2 + Thrust) * 1000 + idle_PWM;
% M2 = ((Pitch - Roll / 2 + Yaw) * Thrust / 2 + Thrust) * 1000 + idle_PWM;
% M3 = ((-Roll - Yaw) * Thrust / 2 + Thrust) * 1000 + idle_PWM;
% M4 = ((-Pitch - Roll / 2 + Yaw) * Thrust / 2 + Thrust) * 1000 + idle_PWM;
% M5 = ((-Pitch + Roll / 2 - Yaw) * Thrust / 2 + Thrust) * 1000 + idle_PWM;
% M6 = ((Roll + Yaw) * Thrust / 2 + Thrust) * 1000 + idle_PWM;
% M7 = 1000;
% M8 = 1000;

% % Hex X (From Adam)
% M1 = uint16(single(((-Roll - Yaw) * Thrust / 3 + Thrust) * single(1000))) + idle_PWM;
% M2 = uint16(single(((Roll + Yaw) * Thrust / 3 + Thrust) * single(1000))) + idle_PWM;
% M3 = uint16(single(((Pitch + (Roll / 2) - Yaw) * Thrust / 3 + Thrust) * single(1000))) + idle_PWM;
% M4 = uint16(single(((-Pitch - (Roll / 2) + Yaw) * Thrust / 3 + Thrust) * single(1000))) + idle_PWM;
% M5 = uint16(single(((Pitch - (Roll / 2) + Yaw) * Thrust / 3 + Thrust) * single(1000))) + idle_PWM;
% M6 = uint16(single(((-Pitch + (Roll / 2) - Yaw) * Thrust / 3 + Thrust) * single(1000))) + idle_PWM;

% Hex X (Version 2)
% Roll/Yaw
% M1 = ((-Roll - Yaw) * Thrust / 2 + Thrust) * 1000 + idle_PWM;
% M2 = ((Roll + Yaw) * Thrust / 2 + Thrust) * 1000 + idle_PWM;
% % + Pitch/Roll
% M6 = ((Pitch + Roll / 2 - Yaw) * Thrust / 2 + Thrust) * 1000 + idle_PWM;
% M4 = ((Pitch - Roll / 2 + Yaw) * Thrust / 2 + Thrust) * 1000 + idle_PWM;
% % - Pitch/Roll
% M5 = ((-Pitch - Roll / 2 + Yaw) * Thrust / 2 + Thrust) * 1000 + idle_PWM;
% M3 = ((-Pitch + Roll / 2 - Yaw) * Thrust / 2 + Thrust) * 1000 + idle_PWM;

== matlab function pixhawkController/Receive_IMU_Data/GPS B2D ==
  data: dvalid input; bytes input; Lat_Degrees output; Lat_Mins output uint16; Lat_Fractions output uint16; Lat_Dir output uint16; Lon_Degrees output uint16; Lon_Mins output uint16; Lon_Fractions output uint16; Lon_Dir output uint16; gps_alt output; gps_alt_fraction output; gps_speed output uint16; gps_speed_fraction output uint16; gps_trackangle output uint16; gps_trackangle_fraction output uint16; gps_date output; gps_month output; gps_year output; gps_time_h output; gps_time_m output; gps_time_s output
function [Lat_Degrees,Lat_Mins,Lat_Fractions,Lat_Dir,Lon_Degrees,Lon_Mins,Lon_Fractions,Lon_Dir,gps_alt, gps_alt_fraction, gps_speed,gps_speed_fraction,gps_trackangle,gps_trackangle_fraction, gps_date, gps_month, gps_year, gps_time_h, gps_time_m, gps_time_s] = B2D(dvalid,bytes)

persistent XLat_Degrees XLat_Mins XLat_Fractions XLat_Dir XLon_Degrees XLon_Mins XLon_Fractions XLon_Dir Xgps_speed Xgps_speed_fraction Xgps_trackangle Xgps_trackangle_fraction Xgps_date Xgps_month Xgps_year Xgps_time_h Xgps_time_m Xgps_time_s Xgps_alt Xgps_alt_fraction

	
% Initialize persistent data
if isempty(XLat_Degrees)
   XLat_Degrees=uint16(0);
end
if isempty(XLat_Mins)
   XLat_Mins=uint16(0);
end
if isempty(XLat_Fractions)
   XLat_Fractions=uint16(0);
end
if isempty(XLat_Dir)
   XLat_Dir=uint16(0);
end
if isempty(XLon_Degrees)
   XLon_Degrees=uint16(0);
end
if isempty(XLon_Mins)
   XLon_Mins=uint16(0);
end
if isempty(XLon_Fractions)
   XLon_Fractions=uint16(0);
end
if isempty(XLon_Dir)
   XLon_Dir=uint16(0);
end
if isempty(Xgps_speed)
   Xgps_speed=uint16(0);
end
if isempty(Xgps_speed_fraction)
   Xgps_speed_fraction=uint16(0);
end
if isempty(Xgps_trackangle)
   Xgps_trackangle=uint16(0);
end
if isempty(Xgps_trackangle_fraction)
   Xgps_trackangle_fraction=uint16(0);
end
if isempty(Xgps_date)
   Xgps_date=uint16(0);
end
if isempty(Xgps_month)
   Xgps_month=uint16(0);
end
if isempty(Xgps_year)
   Xgps_year=uint16(0);
end
if isempty(Xgps_time_h)
   Xgps_time_h=uint16(0);
end
if isempty(Xgps_time_m)
   Xgps_time_m=uint16(0);
end
if isempty(Xgps_time_s)
   Xgps_time_s=uint16(0);
end
if isempty(Xgps_alt)
   Xgps_alt=uint16(0);
end
if isempty(Xgps_alt_fraction)
   Xgps_alt_fraction=uint16(0);
end


% Lat_Degrees = zeros(1,1,'uint16');
% Lat_Mins = zeros(1,1,'uint16');
% Lat_Fractions = zeros(1,1,'uint16');
% Lat_Dir = zeros(1,1,'uint16');
% Lon_Degrees =zeros(1,1,'uint16');
% Lon_Mins = zeros(1,1,'uint16');
% Lon_Fractions = zeros(1,1,'uint16');
% Lon_Dir = zeros(1,1,'uint16');
% gps_speed = zeros(1,1,'uint16');
% gps_speed_fraction = zeros(1,1,'uint16');
% gps_trackangle = zeros(1,1,'uint16');
% gps_trackangle_fraction = zeros(1,1,'uint16');

if (dvalid == 1)
    
  %Lat_Degrees(1)=double(typecast(bytes(2:-1:1),'uint16'));
  
  %Lat_Degrees=[bytes(2); bytes(1)];
    YLat_Degrees= typecast(bytes(2:-1:1),'uint16');
    YLat_Mins= typecast(bytes(4:-1:3),'uint16');
    YLat_Fractions= typecast(bytes(6:-1:5),'uint16');
    YLat_Dir= typecast(bytes(8:-1:7),'uint16');
    YLon_Degrees= typecast(bytes(10:-1:9),'uint16');
    YLon_Mins= typecast(bytes(12:-1:11),'uint16');
    YLon_Fractions= typecast(bytes(14:-1:13),'uint16');
    YLon_Dir= typecast(bytes(16:-1:15),'uint16');
    Ygps_alt= typecast(bytes(18:-1:17),'uint16');
    Ygps_alt_fraction= typecast(bytes(20:-1:19),'uint16');
    Ygps_speed= typecast(bytes(22:-1:21),'uint16');
    Ygps_speed_fraction= typecast(bytes(24:-1:23),'uint16');
    Ygps_trackangle= typecast(bytes(26:-1:25),'uint16');
    Ygps_trackangle_fraction= typecast(bytes(28:-1:27),'uint16');
    Ygps_date= typecast(bytes(30:-1:29),'uint16');
    Ygps_month= typecast(bytes(32:-1:31),'uint16');
    Ygps_year= typecast(bytes(34:-1:33),'uint16');
    Ygps_time_h= typecast(bytes(36:-1:35),'uint16');
    Ygps_time_m= typecast(bytes(38:-1:37),'uint16');
    Ygps_time_s= typecast(bytes(40:-1:39),'uint16');
    
    
    
    XLat_Degrees=YLat_Degrees(1) ;
    XLat_Mins=YLat_Mins(1) ;
    XLat_Fractions=YLat_Fractions(1) ;
    XLat_Dir=YLat_Dir(1);
    XLon_Degrees=YLon_Degrees(1);
    XLon_Mins=YLon_Mins(1);
    XLon_Fractions=YLon_Fractions(1);
    XLon_Dir=YLon_Dir(1);
    Xgps_speed=Ygps_speed(1); 
    Xgps_speed_fraction=Ygps_speed_fraction(1);
    Xgps_trackangle=Ygps_trackangle(1);
    Xgps_trackangle_fraction=Ygps_trackangle_fraction(1);
    Xgps_date=Ygps_date(1);
    Xgps_month=Ygps_month(1);
    Xgps_year=Ygps_year(1);
    Xgps_time_h=Ygps_time_h(1);
    Xgps_time_m=Ygps_time_m(1);
    Xgps_time_s=Ygps_time_s(1);
    Xgps_alt=Ygps_alt(1);
    Xgps_alt_fraction=Ygps_alt_fraction(1);
    
    
end
    
    %ivalue = typecast(bytes(24:-1:23),'uint16');
   Lat_Degrees=XLat_Degrees ;
   Lat_Mins=XLat_Mins ;
   Lat_Fractions=XLat_Fractions ;
   Lat_Dir=XLat_Dir;
   Lon_Degrees=XLon_Degrees;
   Lon_Mins=XLon_Mins;
   Lon_Fractions=XLon_Fractions;
   Lon_Dir=XLon_Dir;
   gps_speed=Xgps_speed; 
   gps_speed_fraction=Xgps_speed_fraction;
   gps_trackangle=Xgps_trackangle;
   gps_trackangle_fraction=Xgps_trackangle_fraction;
   gps_date=Xgps_date;
   gps_month=Xgps_month;
   gps_year=Xgps_year;
   gps_time_h=Xgps_time_h;
   gps_time_m=Xgps_time_m;
   gps_time_s=Xgps_time_s;
   gps_alt=Xgps_alt;
   gps_alt_fraction=Xgps_alt_fraction;
   % value = uint8(ivalue(1));
%end

== matlab function pixhawkController/Receive_IMU_Data/Read Buffer2 ==
  data: dvalid output; imu_data output; bytes input; endinx input; inbuflenSC2 input
function [dvalid, imu_data] = fcn(bytes, endinx, inbuflenSC2)
%inbuflenSC2 length parameter for input buffer

persistent indata inx curinx 


%Constants 
headerlen = 2;
dlen = 40;
cslen = 2;

% Initialize persistent data
if isempty(indata)
    indata = zeros(dlen,1,'uint8');
end
if isempty(inx)
    inx = 1;
end
if isempty(curinx)
    curinx = 1;
end

outbuf = uint8(zeros(dlen,1));

dvalid = uint8(0);
%
while ((endinx ~= 0) && (inx ~= endinx))
    if (curinx == 1)
        if (bytes(inx) == 255) %0xFF
            curinx = curinx + 1;
        else
            curinx=1;
        end       
    elseif (curinx == 2)
        if (bytes(inx) == 251) %0xFB
            curinx = curinx + 1;
        elseif (bytes(inx) == 255) %0xFF
            curinx = 2;
        else
            curinx = 1;
        end
    elseif (curinx == 43)
        if (bytes(inx) == 13) %0x0D
            curinx = curinx + 1;
        else
            curinx = 1;
        end
    elseif (curinx == 44)   % Last data received       
        if (bytes(inx) == 10) %0x0A
            outbuf = indata;    % Copy received data to output buffer            
        %    dvalid = dvalid + uint8(1);         % This data is valid and fresh
            dvalid =uint8(1);         % This data is valid and fresh
        end              
        curinx = 1; % Reset counter             
    else    % Grap Data bytes  
        indata(curinx-headerlen) = bytes(inx);
        curinx = curinx + 1;
    end       
    
    inx = inx + 1;
    if (inx > inbuflenSC2)
        inx = 1;
    end
end

imu_data = outbuf(1:dlen);

== matlab function pixhawkController/Receive_IMU_Data/Read Buffer1 ==
  data: dvalid output; imu_data output; bytes input; endinx input; inbuflenSC2 input
function [dvalid, imu_data] = fcn(bytes, endinx, inbuflenSC2)
%inbuflenSC2 length parameter for input buffer

persistent indata inx curinx 


%Constants 
headerlen = 2;
dlen = 40;
cslen = 2;

% Initialize persistent data
if isempty(indata)
    indata = zeros(dlen,1,'uint8');
end
if isempty(inx)
    inx = 1;
end
if isempty(curinx)
    curinx = 1;
end

outbuf = uint8(zeros(dlen,1));

dvalid = uint8(0);
%
while ((endinx ~= 0) && (inx ~= endinx))
    if (curinx == 1)
        if (bytes(inx) == 255) %0xFF
            curinx = curinx + 1;
        else
            curinx=1;
        end       
    elseif (curinx == 2)
        if (bytes(inx) == 250) %0xFA
            curinx = curinx + 1;
        elseif (bytes(inx) == 255) %0xFF
            curinx = 2;
        else
            curinx = 1;
        end
    elseif (curinx == 43)
        if (bytes(inx) == 13) %0x0D
            curinx = curinx + 1;
        else
            curinx = 1;
        end
    elseif (curinx == 44)   % Last data received       
        if (bytes(inx) == 10) %0x0A
            outbuf = indata;    % Copy received data to output buffer            
        %    dvalid = dvalid + uint8(1);         % This data is valid and fresh
            dvalid =uint8(1);         % This data is valid and fresh
        end              
        curinx = 1; % Reset counter             
    else    % Grap Data bytes  
        indata(curinx-headerlen) = bytes(inx);
        curinx = curinx + 1;
    end       
    
    inx = inx + 1;
    if (inx > inbuflenSC2)
        inx = 1;
    end
end

imu_data = outbuf(1:dlen);
